simulink model "base_model_1_new_Copy"  (R2025b)
settings: Solver=VariableStepAuto  StartTime=0.0  StopTime=3600  RelTol=1e-3
libraries: simulink x2
settings Model: Creator=Gmusl  LastModifiedBy=Gmusl

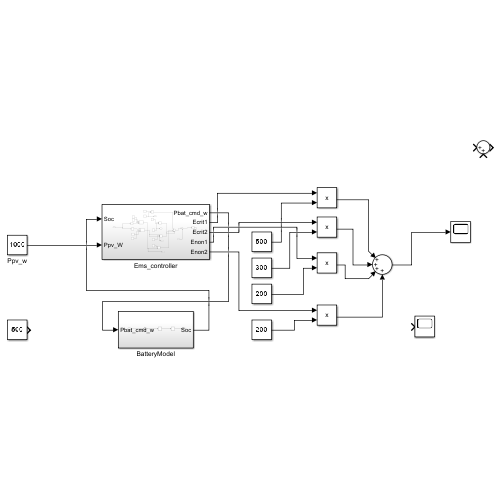
[thumbnail: Simulink's stored preview of the top-level diagram]
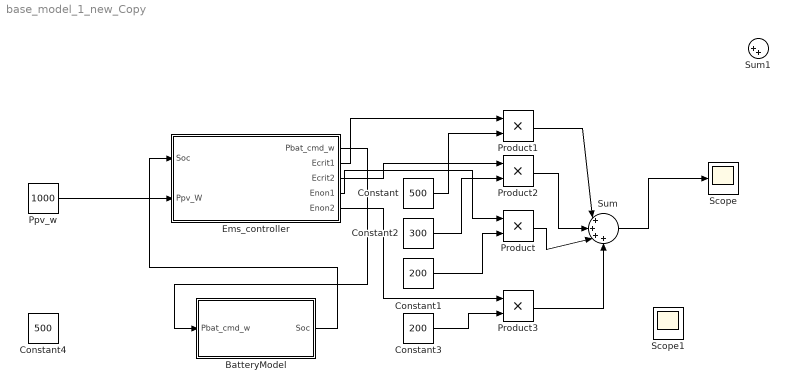
== system base_model_1_new_Copy ==
  BatteryModel : Subsystem
  Constant : Constant  Value=500
  Constant1 : Constant  Value=200
  Constant2 : Constant  Value=300
  Constant3 : Constant  Value=200
  Constant4 : Constant  Value=500
  Ems_controller : Subsystem
  Ppv_w : Constant  Value=1000
  Product{,1..3} (4 alike) : Product
  Scope : Scope
      settings: ActiveDisplayYMinimum=0  ActiveDisplayYMaximum=1
  Scope1 : Scope
      settings: ActiveDisplayYMinimum=-0.47972213353852167  ActiveDisplayYMaximum=1.7031524548434163
  Sum : Sum  Inputs=|++++
  Sum1 : Sum  Inputs=|++
  wires:
  Ppv_w/1 -> Ems_controller/2(Ppv_W)
  Ems_controller/2(Ecrit1) -> Product1/1
  Constant/1 -> Product1/2
  Ems_controller/3(Ecrit2) -> Product2/1
  Constant2/1 -> Product2/2
  Ems_controller/4(Enon1) -> Product/1
  Constant1/1 -> Product/2
  Ems_controller/5(Enon2) -> Product3/1
  Constant3/1 -> Product3/2
  Product1/1 -> Sum/1
  Product2/1 -> Sum/2
  Product/1 -> Sum/3
  Product3/1 -> Sum/4
  Sum/1 -> Scope/1
  BatteryModel/1(Soc) -> Ems_controller/1(Soc)
  Ems_controller/1(Pbat_cmd_w) -> BatteryModel/1(Pbat_cmd_w)

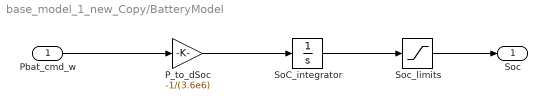
== system base_model_1_new_Copy/BatteryModel ==
  Pbat_cmd_w : Inport
  P_to_dSoc : Gain  Gain=-1/(3.6e6)
  SoC_integrator : Integrator  InitialCondition=0.8
  Soc_limits : Saturate  UpperLimit=0.95  LowerLimit=0.2
  Soc : Outport
  wires:
  Pbat_cmd_w/1 -> P_to_dSoc/1
  P_to_dSoc/1 -> SoC_integrator/1
  SoC_integrator/1 -> Soc_limits/1
  Soc_limits/1 -> Soc/1

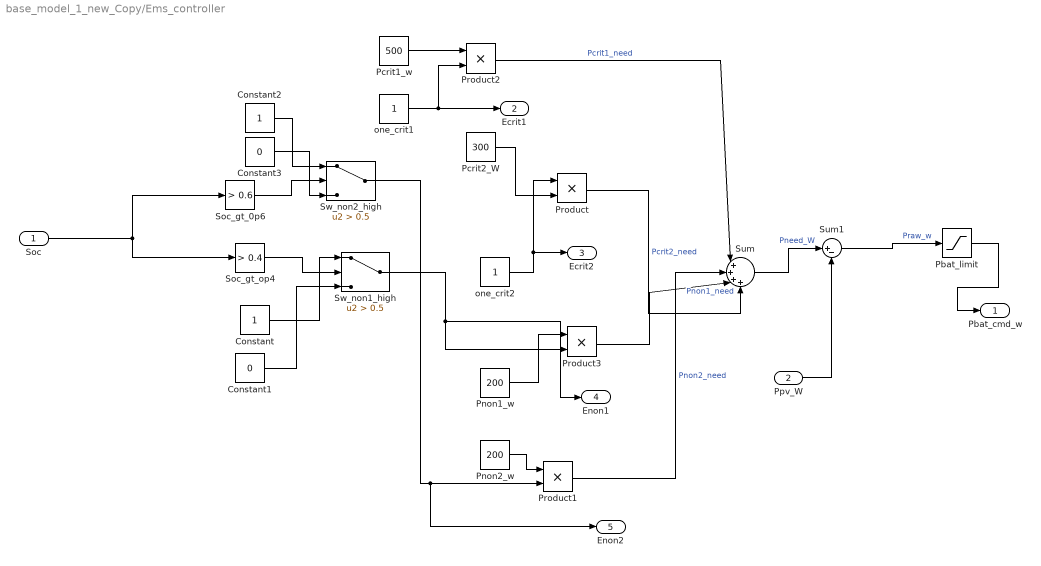
== system base_model_1_new_Copy/Ems_controller ==
  Soc : Inport
  Ppv_W : Inport  Port=2
  Constant : Constant
  Constant1 : Constant  Value=0
  Constant2 : Constant
  Constant3 : Constant  Value=0
  Pbat_limit : Saturate  UpperLimit=2000  LowerLimit=-2000
  Pcrit1_w : Constant  Value=500
  Pcrit2_W : Constant  Value=300
  Pnon1_w : Constant  Value=200
  Pnon2_w : Constant  Value=200
  Product{,1..3} (4 alike) : Product
  Soc_gt_0p6 : simulink/Logic and Bit Operations/Compare To Constant  relop=>  const=0.6  OutDataTypeStr=boolean
  Soc_gt_op4 : simulink/Logic and Bit Operations/Compare To Constant  relop=>  const=0.4  OutDataTypeStr=boolean
  Sum : Sum  Inputs=|++++
  Sum1 : Sum  Inputs=|+-
  Sw_non1_high : Switch  Criteria=u2 > Threshold  Threshold=0.5  SaturateOnIntegerOverflow=off  InputSameDT=off
  Sw_non2_high : Switch  Criteria=u2 > Threshold  Threshold=0.5  SaturateOnIntegerOverflow=off  InputSameDT=off
  one_crit1 : Constant
  one_crit2 : Constant
  Pbat_cmd_w : Outport
  Ecrit1 : Outport  Port=2
  Ecrit2 : Outport  Port=3
  Enon1 : Outport  Port=4
  Enon2 : Outport  Port=5
  wires:
  one_crit1/1 -> Product2/2, Ecrit1/1
  Soc/1 -> Soc_gt_0p6/1, Soc_gt_op4/1
  Soc_gt_op4/1 -> Sw_non1_high/2
  Constant/1 -> Sw_non1_high/1
  Constant1/1 -> Sw_non1_high/3
  Soc_gt_0p6/1 -> Sw_non2_high/2
  Constant3/1 -> Sw_non2_high/3
  Constant2/1 -> Sw_non2_high/1
  Pcrit1_w/1 -> Product2/1
  Product2/1 -> Sum/1  "Pcrit1_need"
  one_crit2/1 -> Product/1, Ecrit2/1
  Pcrit2_W/1 -> Product/2
  Product/1 -> Sum/4  "Pcrit2_need"
  Sw_non1_high/1 -> Enon1/1, Product3/2
  Pnon1_w/1 -> Product3/1
  Product3/1 -> Sum/3  "Pnon1_need"
  Sw_non2_high/1 -> Enon2/1, Product1/2
  Pnon2_w/1 -> Product1/1
  Product1/1 -> Sum/2  "Pnon2_need"
  Sum/1 -> Sum1/1  "Pneed_W"
  Ppv_W/1 -> Sum1/2
  Sum1/1 -> Pbat_limit/1  "Praw_w"
  Pbat_limit/1 -> Pbat_cmd_w/1
